simulink model "MM1MPEG4"  (R2020b)
settings: Solver=VariableStepDiscrete  StartTime=0.0  StopTime=stopTime  FixedStep=0.01  RelTol=1e-3
undefined symbols (not defined in the file or in its folder): m, n
settings Model: Creator=pcuijper  LastModifiedBy=xuanshu
settings SolverCC: ZeroCrossControl=DisableAll
settings DataIOCC: ReturnWorkspaceOutputs=off
settings DebuggingCC: ArithmeticOperatorsInVariantConditions=warning
settings SFSimCC: SimUseLocalCustomCode=off  CustomCodeUndefinedFunction=UseInterfaceOnly
settings RTWCC: RTWUseLocalCustomCode=off
settings CodeAppCC: StateflowObjectComments=on

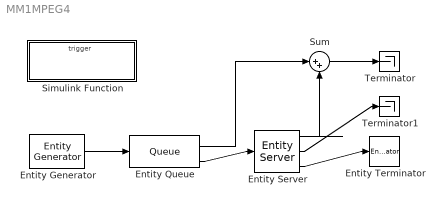
== system MM1MPEG4 ==
  Entity Generator : EntityGenerator  OutputPortMessageModes=m  TimeSource=MATLAB action  IntergenerationTimeAction=|  GenerateEntityAtSimulationStart=off  GenerateAction=|  AttributeName=scene_type|service_time|gene_tstamp|serv_tstamp|over_tstamp  AttributeInitialValue=1|0|0|0|0  EntityType=Structured  EntityTypeName=Entity
      IntergenerationTimeAction=|
      | persistent rngInit;
      | 
      | if isempty(rngInit)
      |     seed = mySeed;
      |     rng(seed);
      |     rngInit = true;
      | end
      | 
      | dt = interArrivalTime;
      GenerateAction=|
      | persistent prev_type;
      | persistent flag;
      | 
      | 
      | if isempty(flag)
      |     prev_type = 1;
      |     flag = [1 1 4 5 1 4];
      | end
      | 
      | event = rand();
      | entity.gene_tstamp = get_curr_time();
      | if prev_type == 1
      |     entity.service_time = 0.020;
      |     if event>0 && event<=0.01
      |         % Scenes = SceneChange
      |         entity.scene_type = 1;
      |         prev_type = 1;
      |     elseif event>0.01 && event<=0.41
      |         % Scene = ActionScene
      |         entity.scene_type = 2;
      |         prev_type = 2;
      |     elseif event>0.41 && event<=0.6
      |         % Scenes = NormalScene
      |         entity.scene_type = 3;
      |         prev_type = 3;
      |     elseif event>0.6 && event<=1
      |         % Scenes = SceneChange
      |         entity.scene_type = 4;
      |         prev_type = 4;
      |     end
      | elseif prev_type == 2
      |     entity.service_time = 0.015;
      |     if event>0 && event<=0.15
      |         % Scenes = SceneChange
      |         entity.scene_type = 1;
      |         prev_type = 1;
      |     elseif event>0.15 && event<=0.95
      |         % Scenes = ActionScene
      |         entity.scene_type = 2;
      |         prev_type = 2;
      |     elseif event>0.95 && event<=1
      |         % Scenes = NormalScene
      |         entity.scene_type = 3;
      |         prev_type = 3;
      |     end
      | elseif prev_type == 3
      |     % Scenes = SceneChange
      |     entity.service_time = 0.010;
      |     if event>0 && event<=0.03
      |         entity.scene_type = 1;
      |         prev_type = 1;
      |         % Scenes = ActionScene
      |     elseif event>0.03 && event<=0.28
      |         entity.scene_type = 2;
      |         prev_type = 2;
      |         % Scenes = NormalScene
      |     elseif event>0.28 && event<=0.98
      |         entity.scene_type = 3;
      |         prev_type = 3;
      |     elseif event>0.98 && event<=1
      |         entity.scene_type = 4;
      |         prev_type = 4;
      |     end
      | elseif prev_type == 4
      |     entity.service_time = 0.005;
      |     % Scenes = SceneChange
      |     if event>0 && event<=0.4
      |         entity.scene_type = 1;
      |         prev_type = 1;
      |     % Scenes = NormalScene
      |     elseif event>0.4 && event<=0.5
      |         entity.scene_type = 3;
      |         prev_type = 3;
      |     % Scenes = QuietScene
      |     elseif event>0.5 && event<=1
      |         entity.scene_type = 4;
      |         prev_type = 4;
      |     end
      | end
  Entity Queue : Queue  InputPortMessageModes=m  OutputPortMessageModes=n,m  Capacity=inf  NumberEntitiesInBlock=on
      settings: OutputPortMap=o1,o5
  Entity Server : EntityServer  InputPortMessageModes=m  OutputPortMessageModes=n,n,m  Capacity=1  ServiceTimeSource=Attribute  ServiceTimeValue=rand(1,1)  ServiceTimeAttributeName=service_time  ServiceTimeAction=|  EntryAction=entity.serv_tstamp = get_curr_time();  ServiceCompleteAction=entity.over_tstamp = get_curr_time();  NumberEntitiesInBlock=on  AverageWait=on
      | persistent rngInit;
      | 
      | if isempty(rngInit)
      |     seed = mySeed+1;
      |     rng(seed);
      |     rngInit = true;
      | end
      | 
      | dt = -interServiceTime * log(1 - rand());
      settings: OutputPortMap=o1,o4,o9
  Entity Terminator : EntityTerminator  InputPortMessageModes=m
  Simulink Function : Subsystem  TreatAsAtomicUnit=on
  Sum : Sum  Inputs=|++
  Terminator : Terminator
  Terminator1 : Terminator
  wires:
  Entity Generator/1 -> Entity Queue/1
  Entity Queue/2 -> Entity Server/1
  Entity Server/3 -> Entity Terminator/1
  Entity Server/1 -> Sum/2
  Entity Queue/1 -> Sum/1
  Sum/1 -> Terminator/1
  Entity Server/2 -> Terminator1/1

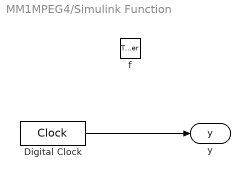
== system MM1MPEG4/Simulink Function ==
  f : TriggerPort  TriggerType=function-call  IsSimulinkFunction=on  FunctionName=get_curr_time  FunctionVisibility=scoped  VariantControl=(inherit)
  Digital Clock : DigitalClock  SampleTime=-1
  y : ArgOut  DisableCoverage=on  ArgumentName=y
  wires:
  Digital Clock/1 -> y/1
